simulink model "Part3_1"  (R2022a)
settings: Solver=VariableStepAuto  StartTime=0.0  StopTime=100  RelTol=1e-3
values from neighbouring files (symbols this model uses):
  D = diag([0.01, 0.01, 0.01])    [Driver33_NL.m]    (also in Driver_3.m; Driver_33.m; Driver_3NL.m)
  g = [0,0,-9.81]    [Driver33_NL.m]    (also in Driver_3.m; Driver_33.m; Driver_3NL.m)
  g2 = [0,0,0,-9.81]    [Driver33_NL.m]    (also in Driver_3.m; Driver_33.m; Driver_3NL.m)
  I_tf = diag([3e-6, 3e-6, 1e-5, 1])    [Driver33_NL.m]    (also in Driver_3.m; Driver_33.m; Driver_3NL.m)
  In = inv(I)    [Driver33_NL.m]    (also in Driver_3.m; Driver_33.m; Driver_3NL.m)
  k = 0.01    [Driver33_NL.m]    (also in Driver_3.m; Driver_33.m; Driver_3NL.m)
  K_d = 1.25    [Driver33_NL.m]    (also in Driver_3.m = 0.943396226415; Driver_33.m = 0.943396226415; Driver_3NL.m = 0.943396226415)
  K_i = 0.1    [Driver33_NL.m]    (also in Driver_3.m = 0.0754716981132; Driver_33.m = 0.0754716981132; Driver_3NL.m = 0.0754716981132)
  K_p = 1    [Driver33_NL.m]    (also in Driver_3.m = 1.9; Driver_33.m = 1.9; Driver_3NL.m = 1.9)
  m = 0.5    [Driver33_NL.m]    (also in Driver_3.m; Driver_33.m; Driver_3NL.m)
  mvec = [1 ... (first row only)    [Driver33_NL.m]    (also in Driver_3.m; Driver_33.m; Driver_3NL.m)
  TF = diag(tf)    [Driver33_NL.m]    (also in Driver_3.m; Driver_33.m)
  TF2 = inv(tf2)    [Driver33_NL.m]    (also in Driver_3.m; Driver_33.m; Driver_3NL.m)
  tf_34 = [L*k, 0, -L*k, 0 ... (first row only)    [Driver33_NL.m]    (also in Driver_3.m; Driver_33.m; Driver_3NL.m)
  w0 = sqrt(9.81*m/(4*k))    [Driver33_NL.m]    (also in Driver_3.m; Driver_33.m; Driver_3NL.m)
settings Model: Creator=askeo  LastModifiedBy=askeo

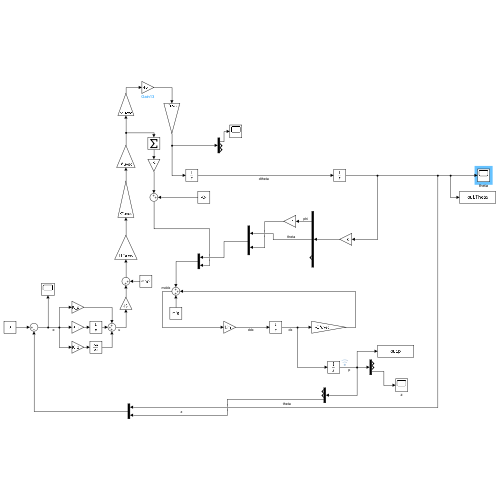
[thumbnail: Simulink's stored preview of the top-level diagram]
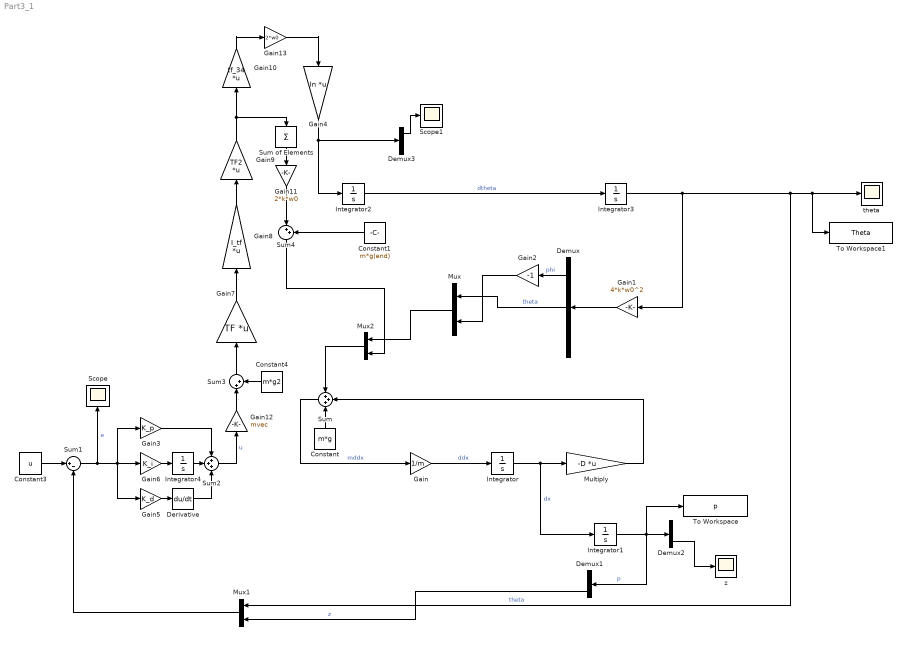
== system Part3_1 ==
  Constant : Constant  Value=m*g
  Constant1 : Constant  Value=m*g(end)
  Constant3 : Constant  Value=u
  Constant4 : Constant  Value=m*g2
  Demux{,1..3} (4 alike) : Demux  Outputs=3
  Derivative : Derivative
  Gain : Gain  Gain=1/m
  Gain1 : Gain  Gain=4*k*w0^2
  Gain10 : Gain  Gain=tf_34  Multiplication=Matrix(K*u) (u vector)
  Gain11 : Gain  Gain=2*k*w0
  Gain12 : Gain  Gain=mvec
  Gain13 : Gain  Gain=2*w0
  Gain2 : Gain  Gain=-1
  Gain3 : Gain  Gain=K_p
  Gain4 : Gain  Gain=In  Multiplication=Matrix(K*u) (u vector)
  Gain5 : Gain  Gain=K_d
  Gain6 : Gain  Gain=K_i
  Gain7 : Gain  Gain=TF  Multiplication=Matrix(K*u) (u vector)
  Gain8 : Gain  Gain=I_tf  Multiplication=Matrix(K*u) (u vector)
  Gain9 : Gain  Gain=TF2  Multiplication=Matrix(K*u) (u vector)
  Integrator : Integrator  InitialCondition=[0;0;0]
  Integrator1 : Integrator  InitialCondition=[0;0;0]
  Integrator2 : Integrator  InitialCondition=[0;0;0]
  Integrator3 : Integrator  InitialCondition=[0; 0; 0]
  Integrator4 : Integrator
  Multiply : Gain  Gain=-D  Multiplication=Matrix(K*u) (u vector)
  Mux : Mux  Inputs=2
  Mux1 : Mux  Inputs=2
  Mux2 : Mux  Inputs=2
  Scope : Scope
  Scope1 : Scope
  Sum : Sum  Inputs=+++
  Sum of Elements : Sum  Inputs=+
  Sum1 : Sum  Inputs=|+-
  Sum2 : Sum  Inputs=+++
  Sum3 : Sum  Inputs=|++
  Sum4 : Sum  Inputs=|++
  To Workspace : ToWorkspace  VariableName=p  SampleTime=-1
  To Workspace1 : ToWorkspace  VariableName=Theta  SampleTime=-1
  theta : Scope
  z : Scope
  wires:
  Gain6/1 -> Integrator4/1
  Constant3/1 -> Sum1/1
  Sum/1 -> Gain/1  "mddx"
  Demux/1 -> Gain2/1  "phi"
  Gain3/1 -> Sum2/1
  Gain1/1 -> Demux/1
  Constant/1 -> Sum/3
  Multiply/1 -> Sum/2
  Gain/1 -> Integrator/1  "ddx"
  Integrator1/1 -> Demux1/1, Demux2/1, To Workspace/1  "p"
  Integrator3/1 -> Gain1/1, Mux1/1, To Workspace1/1, theta/1  "theta"
  Sum1/1 -> Gain5/1, Gain6/1, Gain3/1, Scope/1  "e"
  Gain4/1 -> Integrator2/1, Demux3/1
  Demux/2 -> Mux/1  "theta"
  Gain2/1 -> Mux/2
  Integrator4/1 -> Sum2/2
  Integrator/1 -> Integrator1/1, Multiply/1  "dx"
  Integrator2/1 -> Integrator3/1  "dtheta"
  Gain5/1 -> Derivative/1
  Derivative/1 -> Sum2/3
  Demux1/3 -> Mux1/2  "z"
  Mux1/1 -> Sum1/2
  Constant4/1 -> Sum3/2
  Sum3/1 -> Gain7/1
  Gain7/1 -> Gain8/1
  Gain8/1 -> Gain9/1
  Gain10/1 -> Gain13/1
  Mux/1 -> Mux2/1
  Mux2/1 -> Sum/1
  Constant1/1 -> Sum4/2
  Sum of Elements/1 -> Gain11/1
  Gain11/1 -> Sum4/1
  Sum4/1 -> Mux2/2
  Gain9/1 -> Sum of Elements/1, Gain10/1
  Gain12/1 -> Sum3/1
  Sum2/1 -> Gain12/1  "u"
  Demux2/3 -> z/1
  Demux3/1 -> Scope1/1
  Gain13/1 -> Gain4/1
